simulink library "pbv"  (Simulink 8.1)
settings: Solver=ode45  StartTime=0.0  StopTime=10.0  RelTol=1e-3
undefined symbols (not defined in the file or in its folder): KJUD_AEBConsideredDecel_mps2
libraries: ebdc x1, frdc x1
settings Model: Creator=xsellart  LastModifiedBy=AT015555

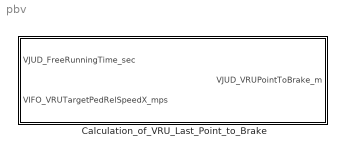
== system pbv ==
  Calculation_of_VRU_Last_Point_to_Brake : Subsystem

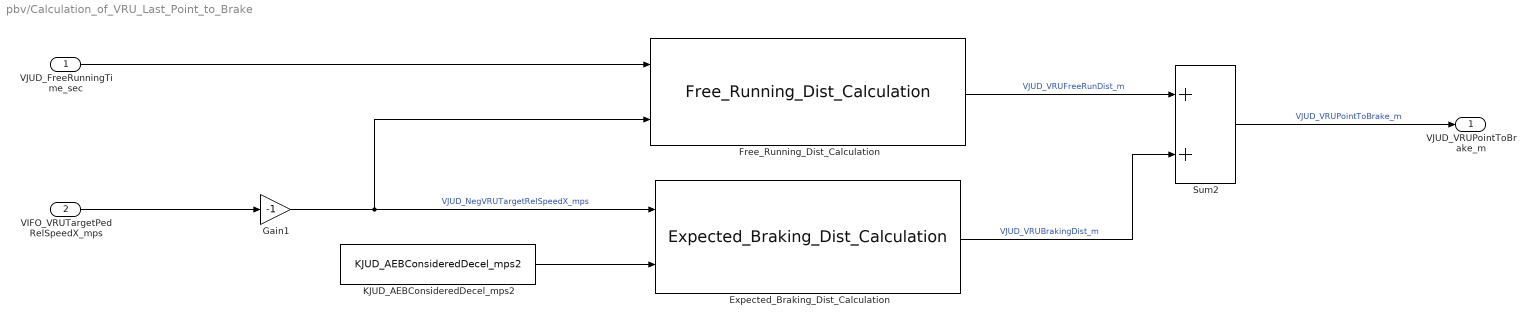
== system pbv/Calculation_of_VRU_Last_Point_to_Brake ==
  VJUD_FreeRunningTime_sec : Inport
  VIFO_VRUTargetPedRelSpeedX_mps : Inport  Port=2
  Expected_Braking_Dist_Calculation : ebdc/Expected_Braking_Dist_Calculation
  Free_Running_Dist_Calculation : frdc/Free_Running_Dist_Calculation
  Gain1 : Gain  Gain=-1  OutDataTypeStr=single
  KJUD_AEBConsideredDecel_mps2 : Constant  Value=KJUD_AEBConsideredDecel_mps2
  Sum2 : Sum
  VJUD_VRUPointToBrake_m : Outport
  wires:
  VJUD_FreeRunningTime_sec/1 -> Free_Running_Dist_Calculation/1
  Expected_Braking_Dist_Calculation/1 -> Sum2/2  "VJUD_VRUBrakingDist_m"
  Free_Running_Dist_Calculation/1 -> Sum2/1  "VJUD_VRUFreeRunDist_m"
  Sum2/1 -> VJUD_VRUPointToBrake_m/1  "VJUD_VRUPointToBrake_m"
  KJUD_AEBConsideredDecel_mps2/1 -> Expected_Braking_Dist_Calculation/2
  Gain1/1 -> Expected_Braking_Dist_Calculation/1, Free_Running_Dist_Calculation/2  "VJUD_NegVRUTargetRelSpeedX_mps"
  VIFO_VRUTargetPedRelSpeedX_mps/1 -> Gain1/1
